simulink model "CRDI_Common_Rail"  (R2019a)
settings: Solver=FixedStepDiscrete  StartTime=0.0  StopTime=10.0  FixedStep=0.001  RelTol=1e-3
settings Model: DataDictionary=CRDI_Common_Rail.sldd  Creator=user  LastModifiedBy=user
settings ConfigComp: DVTestSuiteOptimization=Auto  DVDetectDeadLogic=on  DVDetectOutOfBounds=on  DVRebuildModelRepresentation=Always

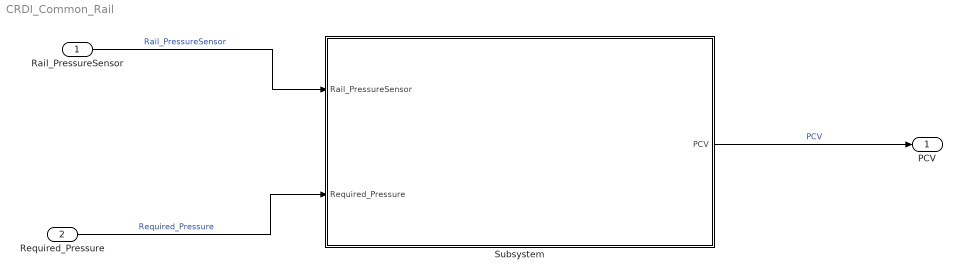
== system CRDI_Common_Rail ==
  Rail_PressureSensor : Inport  OutDataTypeStr=uint16
  Required_Pressure : Inport  Port=2  OutDataTypeStr=uint16
  Subsystem : Subsystem  TreatAsAtomicUnit=on
  PCV : Outport  OutDataTypeStr=boolean
  wires:
  Rail_PressureSensor/1 -> Subsystem/1(Rail_PressureSensor)  "Rail_PressureSensor"
  Required_Pressure/1 -> Subsystem/2(Required_Pressure)  "Required_Pressure"
  Subsystem/1(PCV) -> PCV/1  "PCV"

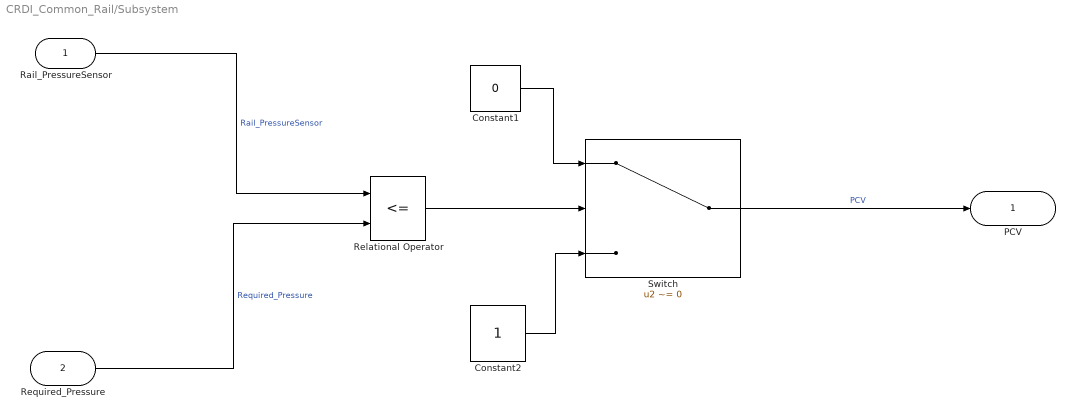
== system CRDI_Common_Rail/Subsystem ==
  Rail_PressureSensor : Inport  OutDataTypeStr=uint16
  Required_Pressure : Inport  Port=2  OutDataTypeStr=uint16
  Constant1 : Constant  Value=0  OutDataTypeStr=uint8
  Constant2 : Constant  OutDataTypeStr=uint8
  Relational Operator : RelationalOperator  Operator=<=  OutDataTypeStr=boolean  RndMeth=Simplest
  Switch : Switch  Criteria=u2 ~= 0  OutDataTypeStr=boolean
  PCV : Outport  OutDataTypeStr=boolean
  wires:
  Required_Pressure/1 -> Relational Operator/2  "Required_Pressure"
  Relational Operator/1 -> Switch/2
  Rail_PressureSensor/1 -> Relational Operator/1  "Rail_PressureSensor"
  Constant1/1 -> Switch/1
  Switch/1 -> PCV/1  "PCV"
  Constant2/1 -> Switch/3
